simulink model "Continu"  (R2025b)
settings: Solver=VariableStepAuto  StartTime=0.0  StopTime=10.0  RelTol=1e-3
undefined symbols (not defined in the file): dspblkCoreblockFVToolHelper, gcbh
settings Model: Creator=elio  LastModifiedBy=elio

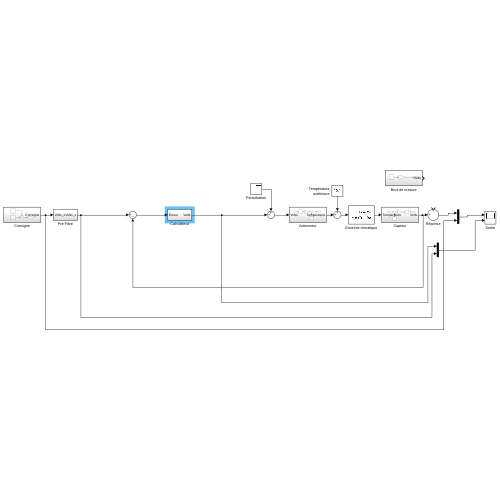
[thumbnail: Simulink's stored preview of the top-level diagram]
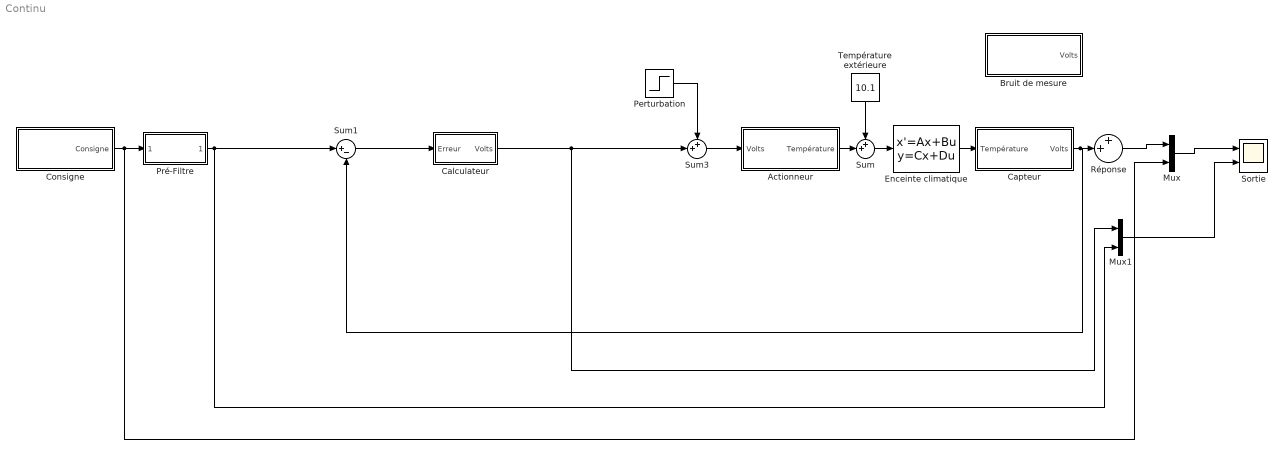
== system Continu ==
  Actionneur : Subsystem
  Bruit de mesure : Subsystem
  Calculateur : Subsystem
  Capteur : Subsystem
  Consigne : Subsystem
  Enceinte climatique : StateSpace  A=-2  B=2  D=0  InitialCondition=9.95
  Mux : Mux  Inputs=2
  Mux1 : Mux  Inputs=2
  Perturbation : Step  Time=2  SampleTime=0.01
  Pré-Filtre : Subsystem
  Réponse : Sum  Inputs=++|
  Sortie : Scope  NumInputPorts=2
      settings: ActiveDisplayYMinimum=0.97433896891638572  ActiveDisplayYMaximum=2.730949279752529
  Sum : Sum  Inputs=++|
  Sum1 : Sum  Inputs=|+-
  Sum3 : Sum  Inputs=++|
  Température extérieure : Constant  Value=10.1
  wires:
  Sum1/1 -> Calculateur/1(Erreur)
  Capteur/1(Volts) -> Sum1/2, Réponse/2
  Température extérieure/1 -> Sum/1
  Réponse/1 -> Mux/1
  Sum/1 -> Enceinte climatique/1
  Consigne/1(Consigne) -> Pré-Filtre/1(Volts_e), Mux/2
  Sum3/1 -> Actionneur/1(Volts)
  Calculateur/1(Volts) -> Sum3/2, Mux1/1
  Mux/1 -> Sortie/1
  Pré-Filtre/1(Volts_s) -> Sum1/1, Mux1/2
  Enceinte climatique/1 -> Capteur/1(Température)
  Actionneur/1(Température) -> Sum/2
  Mux1/1 -> Sortie/2
  Perturbation/1 -> Sum3/1

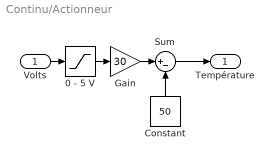
== system Continu/Actionneur ==
  Volts : Inport
  "0 - 5 V " : Saturate  UpperLimit=5  LowerLimit=0
  Constant : Constant  Value=50
  Gain : Gain  Gain=30
  Sum : Sum  Inputs=|+-
  Température : Outport
  wires:
  Volts/1 -> "0 - 5 V "/1
  "0 - 5 V "/1 -> Gain/1
  Gain/1 -> Sum/1
  Constant/1 -> Sum/2
  Sum/1 -> Température/1

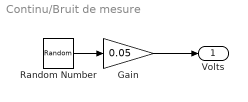
== system Continu/Bruit de mesure ==
  Gain : Gain  Gain=0.05
  Random Number : RandomNumber  Variance=0.5  SampleTime=0.01
  Volts : Outport
  wires:
  Random Number/1 -> Gain/1
  Gain/1 -> Volts/1

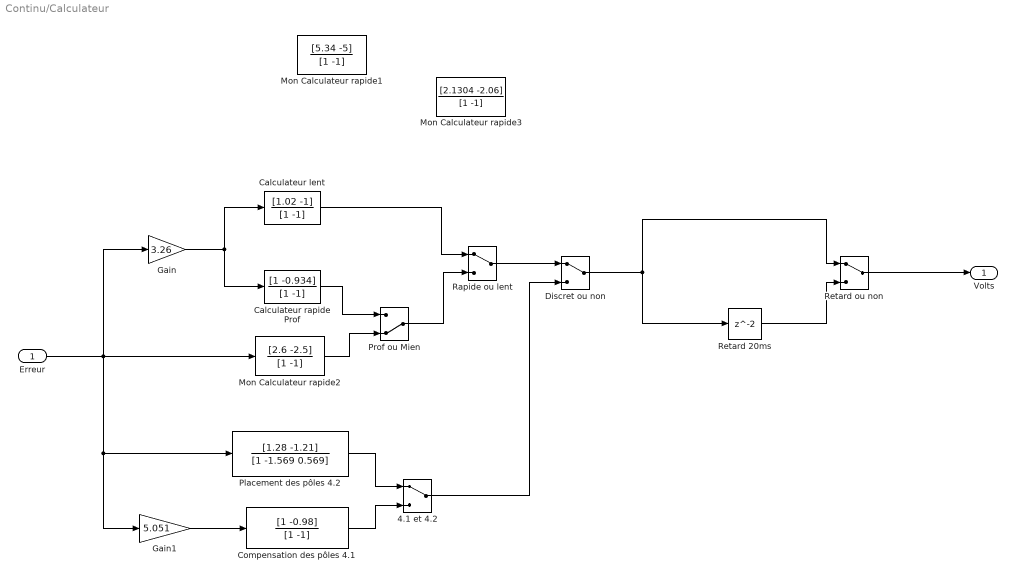
== system Continu/Calculateur ==
  Erreur : Inport
  4.1 et 4.2 : ManualSwitch
  Calculateur lent : DiscreteFilter  LoadFcn=dspblkCoreblockFVToolHelper(gcbh,'load');  Numerator=[1.02 -1]  Denominator=[1 -1]  SampleTime=0.01
      settings: CopyFcn=dspblkCoreblockFVToolHelper(gcbh,'copy');  DeleteFcn=dspblkCoreblockFVToolHelper(gcbh,'close');  ModelCloseFcn=dspblkCoreblockFVToolHelper(gcbh,'close');  PreSaveFcn=dspblkCoreblockFVToolHelper(gcbh,'presave');  PostSaveFcn=dspblkCoreblockFVToolHelper(gcbh,'postsave');  CloseFcn=dspblkCoreblockFVToolHelper(gcbh,'close');
  Calculateur rapide Prof : DiscreteFilter  LoadFcn=dspblkCoreblockFVToolHelper(gcbh,'load');  Numerator=[1 -0.934]  Denominator=[1 -1]  SampleTime=0.01
      settings: CopyFcn=dspblkCoreblockFVToolHelper(gcbh,'copy');  DeleteFcn=dspblkCoreblockFVToolHelper(gcbh,'close');  ModelCloseFcn=dspblkCoreblockFVToolHelper(gcbh,'close');  PreSaveFcn=dspblkCoreblockFVToolHelper(gcbh,'presave');  PostSaveFcn=dspblkCoreblockFVToolHelper(gcbh,'postsave');  CloseFcn=dspblkCoreblockFVToolHelper(gcbh,'close');
  Compensation des pôles 4.1 : DiscreteFilter  LoadFcn=dspblkCoreblockFVToolHelper(gcbh,'load');  Numerator=[1 -0.98]  Denominator=[1 -1]  SampleTime=0.01
      settings: CopyFcn=dspblkCoreblockFVToolHelper(gcbh,'copy');  DeleteFcn=dspblkCoreblockFVToolHelper(gcbh,'close');  ModelCloseFcn=dspblkCoreblockFVToolHelper(gcbh,'close');  PreSaveFcn=dspblkCoreblockFVToolHelper(gcbh,'presave');  PostSaveFcn=dspblkCoreblockFVToolHelper(gcbh,'postsave');  CloseFcn=dspblkCoreblockFVToolHelper(gcbh,'close');
  Discret ou non : ManualSwitch
  Gain : Gain  Gain=3.26
  Gain1 : Gain  Gain=5.051
  Mon Calculateur rapide1 : DiscreteFilter  LoadFcn=dspblkCoreblockFVToolHelper(gcbh,'load');  Numerator=[5.34 -5]  Denominator=[1 -1]  SampleTime=0.01
      settings: CopyFcn=dspblkCoreblockFVToolHelper(gcbh,'copy');  DeleteFcn=dspblkCoreblockFVToolHelper(gcbh,'close');  ModelCloseFcn=dspblkCoreblockFVToolHelper(gcbh,'close');  PreSaveFcn=dspblkCoreblockFVToolHelper(gcbh,'presave');  PostSaveFcn=dspblkCoreblockFVToolHelper(gcbh,'postsave');  CloseFcn=dspblkCoreblockFVToolHelper(gcbh,'close');
  Mon Calculateur rapide2 : DiscreteFilter  LoadFcn=dspblkCoreblockFVToolHelper(gcbh,'load');  Numerator=[2.6 -2.5]  Denominator=[1 -1]  SampleTime=0.01
      settings: CopyFcn=dspblkCoreblockFVToolHelper(gcbh,'copy');  DeleteFcn=dspblkCoreblockFVToolHelper(gcbh,'close');  ModelCloseFcn=dspblkCoreblockFVToolHelper(gcbh,'close');  PreSaveFcn=dspblkCoreblockFVToolHelper(gcbh,'presave');  PostSaveFcn=dspblkCoreblockFVToolHelper(gcbh,'postsave');  CloseFcn=dspblkCoreblockFVToolHelper(gcbh,'close');
  Mon Calculateur rapide3 : DiscreteFilter  LoadFcn=dspblkCoreblockFVToolHelper(gcbh,'load');  Numerator=[2.1304 -2.06]  Denominator=[1 -1]  SampleTime=0.01
      settings: CopyFcn=dspblkCoreblockFVToolHelper(gcbh,'copy');  DeleteFcn=dspblkCoreblockFVToolHelper(gcbh,'close');  ModelCloseFcn=dspblkCoreblockFVToolHelper(gcbh,'close');  PreSaveFcn=dspblkCoreblockFVToolHelper(gcbh,'presave');  PostSaveFcn=dspblkCoreblockFVToolHelper(gcbh,'postsave');  CloseFcn=dspblkCoreblockFVToolHelper(gcbh,'close');
  Placement des pôles 4.2 : DiscreteFilter  LoadFcn=dspblkCoreblockFVToolHelper(gcbh,'load');  Numerator=[1.28 -1.21]  Denominator=[1 -1.569 0.569]  SampleTime=0.01
      settings: CopyFcn=dspblkCoreblockFVToolHelper(gcbh,'copy');  DeleteFcn=dspblkCoreblockFVToolHelper(gcbh,'close');  ModelCloseFcn=dspblkCoreblockFVToolHelper(gcbh,'close');  PreSaveFcn=dspblkCoreblockFVToolHelper(gcbh,'presave');  PostSaveFcn=dspblkCoreblockFVToolHelper(gcbh,'postsave');  CloseFcn=dspblkCoreblockFVToolHelper(gcbh,'close');
  Prof ou Mien : ManualSwitch  CurrentSetting=0
  Rapide ou lent : ManualSwitch
  Retard 20ms : Delay  InitialCondition=0  SampleTime=0.01
  Retard ou non : ManualSwitch
  Volts : Outport
  wires:
  Erreur/1 -> Mon Calculateur rapide2/1, Gain/1, Gain1/1, Placement des pôles 4.2/1
  Calculateur lent/1 -> Rapide ou lent/1
  Gain/1 -> Calculateur rapide Prof/1, Calculateur lent/1
  Mon Calculateur rapide2/1 -> Prof ou Mien/2
  Calculateur rapide Prof/1 -> Prof ou Mien/1
  Prof ou Mien/1 -> Rapide ou lent/2
  Rapide ou lent/1 -> Discret ou non/1
  Gain1/1 -> Compensation des pôles 4.1/1
  Compensation des pôles 4.1/1 -> 4.1 et 4.2/2
  Placement des pôles 4.2/1 -> 4.1 et 4.2/1
  4.1 et 4.2/1 -> Discret ou non/2
  Discret ou non/1 -> Retard ou non/1, Retard 20ms/1
  Retard ou non/1 -> Volts/1
  Retard 20ms/1 -> Retard ou non/2

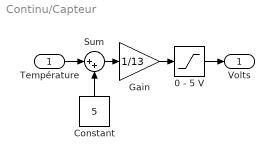
== system Continu/Capteur ==
  Température : Inport
  "0 - 5 V " : Saturate  UpperLimit=5  LowerLimit=0
  Constant : Constant  Value=5
  Gain : Gain  Gain=1/13
  Sum : Sum  Inputs=|++
  Volts : Outport
  wires:
  Constant/1 -> Sum/2
  Température/1 -> Sum/1
  Sum/1 -> Gain/1
  Gain/1 -> "0 - 5 V "/1
  "0 - 5 V "/1 -> Volts/1

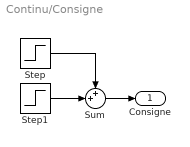
== system Continu/Consigne ==
  Step : Step  Time=4  After=-0.5  SampleTime=0.01
  Step1 : Step  Time=0.5  Before=1.66  After=2.33  SampleTime=0.01
  Sum : Sum  Inputs=++|
  Consigne : Outport
  wires:
  Step/1 -> Sum/1
  Step1/1 -> Sum/2
  Sum/1 -> Consigne/1

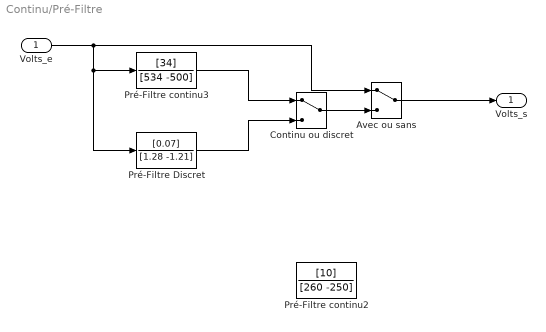
== system Continu/Pré-Filtre ==
  Volts_e : Inport
  Avec ou sans : ManualSwitch
  Continu ou discret : ManualSwitch
  Pré-Filtre Discret : DiscreteFilter  LoadFcn=dspblkCoreblockFVToolHelper(gcbh,'load');  Numerator=[0.07]  Denominator=[1.28 -1.21]  SampleTime=0.01
      settings: CopyFcn=dspblkCoreblockFVToolHelper(gcbh,'copy');  DeleteFcn=dspblkCoreblockFVToolHelper(gcbh,'close');  ModelCloseFcn=dspblkCoreblockFVToolHelper(gcbh,'close');  PreSaveFcn=dspblkCoreblockFVToolHelper(gcbh,'presave');  PostSaveFcn=dspblkCoreblockFVToolHelper(gcbh,'postsave');  CloseFcn=dspblkCoreblockFVToolHelper(gcbh,'close');
  Pré-Filtre continu2 : DiscreteFilter  LoadFcn=dspblkCoreblockFVToolHelper(gcbh,'load');  Numerator=[10]  Denominator=[260 -250]  SampleTime=0.01
      settings: CopyFcn=dspblkCoreblockFVToolHelper(gcbh,'copy');  DeleteFcn=dspblkCoreblockFVToolHelper(gcbh,'close');  ModelCloseFcn=dspblkCoreblockFVToolHelper(gcbh,'close');  PreSaveFcn=dspblkCoreblockFVToolHelper(gcbh,'presave');  PostSaveFcn=dspblkCoreblockFVToolHelper(gcbh,'postsave');  CloseFcn=dspblkCoreblockFVToolHelper(gcbh,'close');
  Pré-Filtre continu3 : DiscreteFilter  LoadFcn=dspblkCoreblockFVToolHelper(gcbh,'load');  Numerator=[34]  Denominator=[534 -500]  SampleTime=0.01
      settings: CopyFcn=dspblkCoreblockFVToolHelper(gcbh,'copy');  DeleteFcn=dspblkCoreblockFVToolHelper(gcbh,'close');  ModelCloseFcn=dspblkCoreblockFVToolHelper(gcbh,'close');  PreSaveFcn=dspblkCoreblockFVToolHelper(gcbh,'presave');  PostSaveFcn=dspblkCoreblockFVToolHelper(gcbh,'postsave');  CloseFcn=dspblkCoreblockFVToolHelper(gcbh,'close');
  Volts_s : Outport
  wires:
  Volts_e/1 -> Pré-Filtre continu3/1, Pré-Filtre Discret/1, Avec ou sans/1
  Avec ou sans/1 -> Volts_s/1
  Pré-Filtre continu3/1 -> Continu ou discret/1
  Continu ou discret/1 -> Avec ou sans/2
  Pré-Filtre Discret/1 -> Continu ou discret/2
